simulink model "vipcellcounting"  (R2015b)
settings: Solver=FixedStepDiscrete  StartTime=0.0  StopTime=inf  RelTol=1e-3
undefined symbols (not defined in the file or in its folder): gray, strel
libraries: visiontextngfix x3, visionmorphops x2, visionstatistics x1, simulink x1, visionsinks x1, vipmisc x1, visionconversions x1, dspvision x1
settings Model: FPTRunName=Active  ExtModeAutoUpdateStatusClock=off  Creator=The MathWorks, Inc.  LastModifiedBy=The MathWorks, Inc.
settings DataIOCC: SaveFormat=Array  SaveOutput=off  SignalLogging=off  SaveTime=off
settings OptimizationCC: ExpressionDepthLimit=2147483647  InitFltsAndDblsToZero=on  BufferReusableBoundary=off
settings DebuggingCC: UnderspecifiedInitializationDetection=Classic  MergeDetectMultiDrivingBlocksExec=none  SignalResolutionControl=TryResolveAllWithWarning  SolverPrmCheckMsg=warning  MultiTaskDSMMsg=warning  MultiTaskCondExecSysMsg=none  FcnCallInpInsideContextMsg=UseLocalSettings  BusObjectLabelMismatch=none  StateNameClashWarn=warning  StrictBusMsg=None
settings HardwareCC: ProdBitPerPointer=32  ProdLargestAtomicFloat=None  ProdIntDivRoundTo=Undefined  ProdEndianess=Unspecified  ProdWordSize=32  ProdHWDeviceType=32-bit Generic  TargetBitPerLong=64  TargetBitPerPointer=64  TargetLongLongMode=on  TargetIntDivRoundTo=Zero  TargetEndianess=LittleEndian  TargetWordSize=64  TargetHWDeviceType=Generic->MATLAB Host Computer  ProdEqTarget=off
settings GRTTargetCC: TargetFcnLib=ansi_tfl_tmw_new.mat  GeneratePreprocessorConditionals=Disable all  CombineOutputUpdateFcns=off  GRTInterface=on
settings ConfigComp: CovModelRefEnable=Off

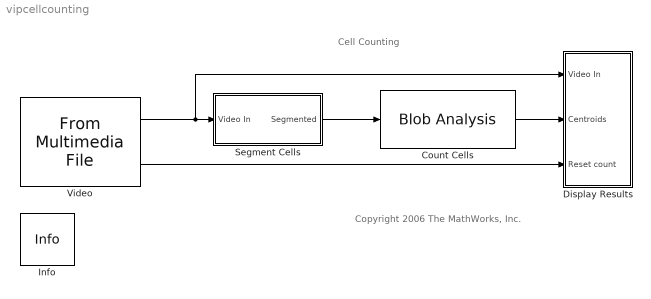
== system vipcellcounting ==
  note: Cell Counting
  note: Copyright 2006 The MathWorks, Inc.
  Count Cells : visionstatistics/Blob Analysis  Tag=vipblks_row_conv  area=off  centroid=on  bBox=off  majorAxis=off  minorAxis=off  angle=off  eccentricity=off  equivDiameterSq=off  extent=off  perimeter=off  maxBlobs=1500  warnIfNumBlobsExceeded=on  isCount=off  useMinArea=on  minArea=7  useMaxArea=on  maxArea=300  excludeBorderBlob=off  outDT=single  isOutVarDim=on  isFill=on  fillValues=-10  conn=8  isLabel=off  outputMode=Binary point scaling  outputWordLength=32  outputFracLength=0  firstCoeffMode=Binary point scaling  firstCoeffWordLength=16  firstCoeffFracLength=14  secondCoeffMode=Binary point scaling  secondCoeffWordLength=32  secondCoeffFracLength=16  accumMode=Binary point scaling  accumWordLength=32  accumFracLength=0  prodOutputMode=Binary point scaling  prodOutputWordLength=32  prodOutputFracLength=16  roundingMode=Floor  overflowMode=off
  Display Results : Subsystem
  Info : vipmisc/Info  SystemSampleTime=-1
  Segment Cells : Subsystem
  Video : dspvision/From Multimedia File  inputFilename=ecolicells.avi  loop=on  numPlays=inf  outputStreams=Video only  videoDataType=single  audioDataType=int16  inheritSampleTime=off  userDefinedSampleTime=1/30  noAudioOutput=off  isIntensityVideo=off  fourcc=Intensity  colorVideoFormat=Separate color signals  outputEOF=on  dataOrg=Column-major  audioFrameSize=1024  computeAudioFrameSize=off  outSamplingMode=Frame based
  wires:
  Video/1 -> Display Results/1(Video In), Segment Cells/1(Video In)
  Video/2 -> Display Results/3(Reset count)
  Count Cells/1 -> Display Results/2(Centroids)
  Segment Cells/1(Segmented) -> Count Cells/1

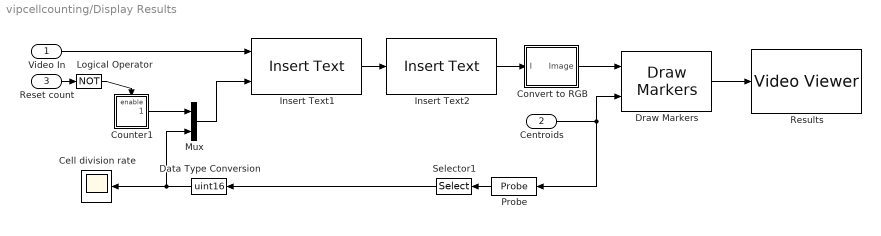
== system vipcellcounting/Display Results ==
  Video In : Inport
  Centroids : Inport  Port=2
  Reset count : Inport  Port=3
  Cell division rate : Scope
  Convert to RGB : Subsystem
  Counter1 : Subsystem  TreatAsAtomicUnit=on
  Data Type Conversion : DataTypeConversion  OutDataTypeStr=uint16
  Draw Markers : visiontextngfix/Draw Markers  shape=Star  size=3  fill=off  fillClrSource=Specify via dialog  display=User-specified value  intensity=155  color=[0 1 0]  opacity=0  viewport=Entire image  antialiasing=off  inType=Obsolete  imagePorts=One multidimensional signal  prodOutputMode=Binary point scaling  prodOutputWordLength=32  prodOutputFracLength=14  memoryMode=Specify word length  memoryWordLength=16  memoryFracLength=15  roundingMode=Floor  overflowMode=off
  Insert Text1 : visiontextngfix/Insert Text  inputType=Obsolete  theText='Frame %d, Count %d'  getTextLocFrom=Specify via dialog  textLoc=[10 10]  getTextColorFrom=Specify via dialog  textColor=1  getTextIntensityFrom=Specify via dialog  textIntensity=1  getTextOpacityFrom=Specify via dialog  textOpacity=1.0  dummyVar2=0  dummyVar3=0  dummyVar4=0  imagePorts=One multidimensional signal  isInputTransposed=off  fontFace=LucidaTypewriterRegular  dummyVar1=0  blockFontSize=16  antiAliased=on
  Insert Text2 : visiontextngfix/Insert Text  inputType=Obsolete  theText='Data set courtesy of Jonathan Young and Michael Elowitz, California Institute of Technology'  getTextLocFrom=Specify via dialog  textLoc=[1 417]  getTextColorFrom=Specify via dialog  textColor=1  getTextIntensityFrom=Specify via dialog  textIntensity=1  getTextOpacityFrom=Specify via dialog  textOpacity=1.0  dummyVar2=0  dummyVar3=0  dummyVar4=0  imagePorts=One multidimensional signal  isInputTransposed=off  fontFace=LucidaSansRegular  dummyVar1=0  blockFontSize=12  antiAliased=on
  Logical Operator : Logic  Operator=NOT  AllPortsSameDT=off  OutDataTypeStr=boolean
  Mux : Mux  Inputs=2
  Probe : Probe  ProbeWidth=off  ProbeSampleTime=off  ProbeComplexSignal=off  ProbeSignalDimensions=on  ProbeWidthDataType=uint8
  Results : visionsinks/Video Viewer  inputType=Obsolete7b  imagePorts=One multidimensional signal  useColorMap=off  colormapValue=gray(256)  specRange=off  minInputVal=0  maxInputVal=255  FigPos=[138 679 534 459]  AxisZoom=on  trueSizedOnce=on  OpenAtMdlStart=on  DefaultConfigurationName=vipscopes.VideoViewerScopeCfg
  Selector1 : Selector  NumberOfDimensions=2  InputPortWidth=3  IndexOptions=Index vector (dialog),Index vector (dialog)  Indices=1,1  OutputSizes=99,1
  wires:
  Video In/1 -> Insert Text1/1
  Mux/1 -> Insert Text1/2
  Insert Text1/1 -> Insert Text2/1
  Draw Markers/1 -> Results/1
  Centroids/1 -> Draw Markers/2, Probe/1
  Insert Text2/1 -> Convert to RGB/1(I)
  Convert to RGB/1(Image) -> Draw Markers/1
  Probe/1 -> Selector1/1
  Selector1/1 -> Data Type Conversion/1
  Data Type Conversion/1 -> Mux/2, Cell division rate/1
  Counter1/1(Out1) -> Mux/1
  Reset count/1 -> Logical Operator/1
  Logical Operator/1 -> Counter1/Enable

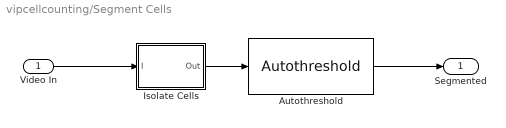
== system vipcellcounting/Segment Cells ==
  Video In : Inport
  Autothreshold : visionconversions/Autothreshold  operator=<=  threshOut=off  effMetricOut=off  userDefinedRange=off  umin=0  umax=1  outOfRngOpt=Warn and saturate  scaleThreshold=on  scaleFactor=single(0.8)  P1Mode=Specify word length  P1WordLength=32  P1FracLength=30  P2Mode=Specify word length  P2WordLength=32  P2FracLength=22  P3Mode=Specify word length  P3WordLength=32  P3FracLength=14  P4Mode=Binary point scaling  P4WordLength=32  P4FracLength=15  Q1Mode=Specify word length  Q1WordLength=32  Q1FracLength=16  EMMode=Specify word length  EMWordLength=16  EMFracLength=14  roundingMode=Floor  overflowMode=off
  Isolate Cells : Subsystem
  Segmented : Outport
  wires:
  Video In/1 -> Isolate Cells/1(I)
  Isolate Cells/1(Out) -> Autothreshold/1
  Autothreshold/1 -> Segmented/1

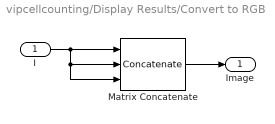
== system vipcellcounting/Display Results/Convert to RGB ==
  I : Inport
  Matrix Concatenate : Concatenate  NumInputs=3  Mode=Multidimensional array  ConcatenateDimension=3
  Image : Outport
  wires:
  Matrix Concatenate/1 -> Image/1
  I/1 -> Matrix Concatenate/3, Matrix Concatenate/2, Matrix Concatenate/1

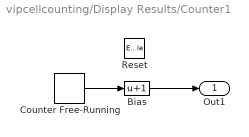
== system vipcellcounting/Display Results/Counter1 ==
  Reset : EnablePort  StatesWhenEnabling=reset
  Bias : Bias  Bias=1
  Counter Free-Running : simulink/Sources/Counter Free-Running  NumBits=16  tsamp=1/30
  Out1 : Outport
  wires:
  Counter Free-Running/1 -> Bias/1
  Bias/1 -> Out1/1

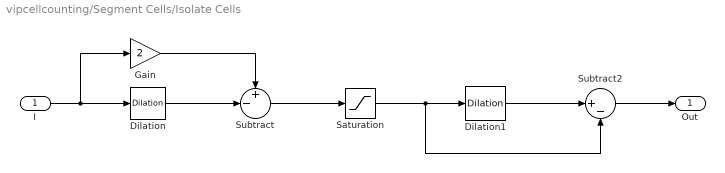
== system vipcellcounting/Segment Cells/Isolate Cells ==
  I : Inport
  Dilation : visionmorphops/Dilation  nhoodsrc=Specify via dialog  strel=strel('square',7)
  Dilation1 : visionmorphops/Dilation  nhoodsrc=Specify via dialog  strel=strel('square',7)
  Gain : Gain  Gain=2
  Saturation : Saturate  UpperLimit=1  LowerLimit=0
  Subtract : Sum  Inputs=+-|  SaturateOnIntegerOverflow=on
  Subtract2 : Sum  Inputs=|+-  SaturateOnIntegerOverflow=on
  Out : Outport
  wires:
  Subtract2/1 -> Out/1
  I/1 -> Dilation/1, Gain/1
  Subtract/1 -> Saturation/1
  Dilation1/1 -> Subtract2/1
  Saturation/1 -> Dilation1/1, Subtract2/2
  Dilation/1 -> Subtract/2
  Gain/1 -> Subtract/1
